simulink model "TBCC_Dyn_Template"  (Simulink 10.0)
settings: Solver=ode4  StartTime=0.0  StopTime=MWS.in.SimTime  FixedStep=MWS.Solve.T  RelTol=1e-3  EnableMultiTasking=on
undefined symbols (not defined in the file or in its folder): stripchar_TMATS
undefined symbols (not defined in the file): MWS
libraries: Lib_Solve_ModelSource_TMATS x2, Lib_Turbo_Ambient_TMATS x1, Lib_Turbo_Burner_TMATS x1, Lib_Turbo_Compressor_TMATS x1, Lib_Turbo_Duct_TMATS x1, Lib_Turbo_Inlet_TMATS x1, Lib_Turbo_Nozzle_TMATS x1, Lib_Turbo_Shaft_TMATS x1, Lib_Turbo_Turbine_TMATS x1, Lib_Solve_IterNRSolverJC_TMATS x1, Lib_Cntrl_FirstOrderSensor_TMATS x1, Lib_Solve_OuterLoopIntegrator_TMATS x1
CloseFcn:
  | run(strcat(MWS.top_level, filesep,'GasTurbine_Dyn_Example_cleanup'))
settings Model: Creator=jwchapm2  LastModifiedBy=Administrator
settings DataIOCC: LimitDataPoints=on  SignalLoggingName=SimulationOutput
settings OptimizationCC: BlockReduction=off  DefaultParameterBehavior=Inlined  BufferReuse=off  ExpressionDepthLimit=2147483647
settings DebuggingCC: SolverPrmCheckMsg=warning  StateNameClashWarn=warning
settings GRTTargetCC: GeneratePreprocessorConditionals=Disable all  CombineOutputUpdateFcns=on  GRTInterface=off
settings ConfigComp: CovExternalEMLEnable=off

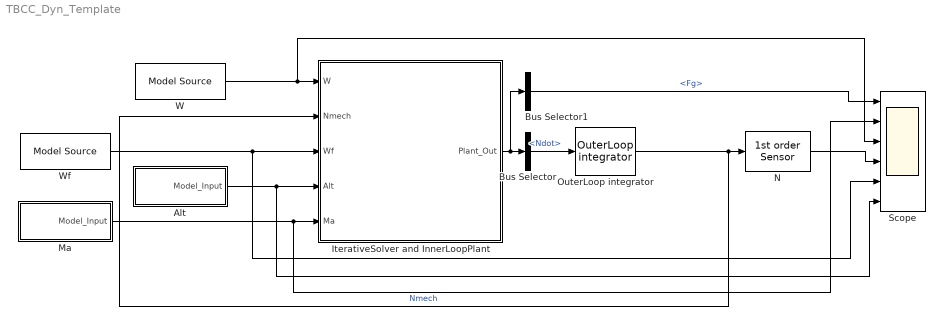
== system TBCC_Dyn_Template ==
  Alt : Subsystem  AncestorBlock=Lib_Solve_ModelSource_TMATS/Model Source  mask(T-MATS: Model Source Library Block){T_vec_M=MWS.in.t_vec, input_array_M=MWS.in.Alt}
      mask prompts: T_vec_M "T_vec_M - Time Vector (x-axis)"; input_array_M "input_array_M - Input Array 1-D ( f(Time))"
      mask help:
      | This block sets up the interface to change simulation variable dynamically.
      | Enter an input vector and time vector to allocate when each element
      | of the intput vector will occur.
      mask Help: web(which('Solver_TMATS_MS.html'),'-helpbrowser')
  Bus Selector : BusSelector  OutputSignals=PlantBus.Ndot
  Bus Selector1 : BusSelector  OutputSignals=PlantBus.Fg
  IterativeSolver and InnerLoopPlant : Subsystem
  Ma : Subsystem  AncestorBlock=Lib_Solve_ModelSource_TMATS/Model Source  mask(T-MATS: Model Source Library Block){T_vec_M=MWS.in.t_vec, input_array_M=MWS.in.Alt}
      mask prompts: T_vec_M "T_vec_M - Time Vector (x-axis)"; input_array_M "input_array_M - Input Array 1-D ( f(Time))"
      mask help:
      | This block sets up the interface to change simulation variable dynamically.
      | Enter an input vector and time vector to allocate when each element
      | of the intput vector will occur.
      mask Help: web(which('Solver_TMATS_MS.html'),'-helpbrowser')
  N : Lib_Cntrl_FirstOrderSensor_TMATS/1st order  Sensor  IC_M=MWS.Solve.N_IC  Sen_Max_M=20000  Sen_Min_M=0  Gain_M=1  Tau_M=0.05  GN_EN_M=off  GN_NST_M=MWS.Solve.T  GN_C_M=1  GN_MinNoise_M=0.3  F_Gain_M=1  F_Drift_M=0
  OuterLoop integrator : Lib_Solve_OuterLoopIntegrator_TMATS/OuterLoop integrator  OL_IC_M=MWS.Solve.N_IC
  Scope : Scope  NumInputPorts=6
  W : Lib_Solve_ModelSource_TMATS/Model Source  T_vec_M=MWS.in.t_vec  input_array_M=MWS.in.Alt
  Wf : Lib_Solve_ModelSource_TMATS/Model Source  T_vec_M=MWS.in.t_vec  input_array_M=MWS.in.Wf
  wires:
  IterativeSolver and InnerLoopPlant/1(Plant_Out) -> Bus Selector1/1, Bus Selector/1
  Bus Selector/1 -> OuterLoop integrator/1  "<Ndot>"
  OuterLoop integrator/1 -> N/1, IterativeSolver and InnerLoopPlant/2(Nmech)  "Nmech"
  Alt/1(Model_Input) -> Scope/6, IterativeSolver and InnerLoopPlant/4(Alt)
  Wf/1 -> Scope/5, IterativeSolver and InnerLoopPlant/3(Wf)
  W/1 -> Scope/3, IterativeSolver and InnerLoopPlant/1(W)
  Bus Selector1/1 -> Scope/1  "<Fg>"
  Ma/1(Model_Input) -> Scope/2, IterativeSolver and InnerLoopPlant/5(Ma)
  N/1 -> Scope/4

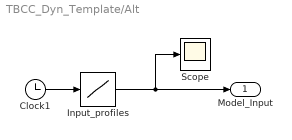
== system TBCC_Dyn_Template/Alt ==
  Clock1 : Clock
      settings: Decimation=100
  Input_profiles : Lookup  InputValues=T_vec_M  Table=input_array_M
  Scope : Scope
  Model_Input : Outport
  wires:
  Clock1/1 -> Input_profiles/1
  Input_profiles/1 -> Scope/1, Model_Input/1

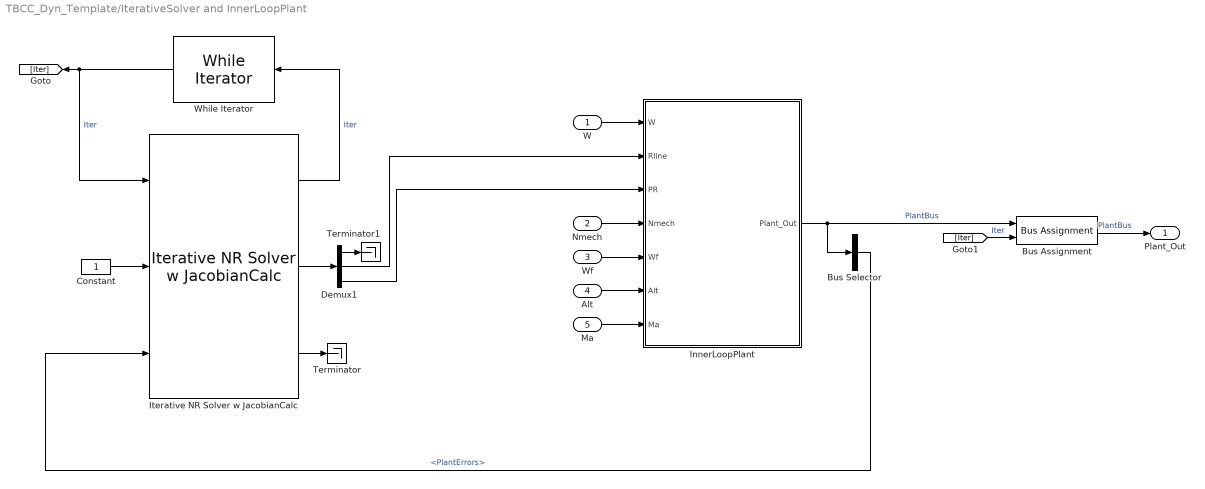
== system TBCC_Dyn_Template/IterativeSolver and InnerLoopPlant ==
  W : Inport
  Nmech : Inport  Port=2
  Wf : Inport  Port=3
  Alt : Inport  Port=4
  Ma : Inport  Port=5
  Bus Assignment : BusAssignment  AssignedSignals=PlantBus.Iter
  Bus Selector : BusSelector  OutputSignals=PlantErrors
  Constant : Constant
  Demux1 : Demux  Outputs=3
  InnerLoopPlant : Subsystem
  Iterative NR Solver w JacobianCalc : Lib_Solve_IterNRSolverJC_TMATS/Iterative NR Solver w JacobianCalc  SJac_Per_M=MWS.Solve.J_Calc_Per  SNR_IC_M=MWS.Solve.NR_IC  SNR_DX_M=MWS.Solve.NR_dx  SNR_Mx_M=100000  SNR_Mn_M=0.0001  SJacobianAttempts_M=MWS.Solve.NR_Jac_Re  Cond_Limits_M=MWS.Solve.C_Lim
  Terminator : Terminator
  Terminator1 : Terminator
  While Iterator : WhileIterator  MaxIters=MWS.Solve.Max_Iter  WhileBlockType=do-while  ShowIterationPort=on
  Plant_Out : Outport
  wires:
  Bus Selector/1 -> Iterative NR Solver w JacobianCalc/3  "<PlantErrors>"
  While Iterator/1 -> [Iter], Iterative NR Solver w JacobianCalc/1  "Iter"
  InnerLoopPlant/1(Plant_Out) -> Bus Selector/1, Bus Assignment/1  "PlantBus"
  Iterative NR Solver w JacobianCalc/1 -> While Iterator/1  "Iter"
  Iterative NR Solver w JacobianCalc/3 -> Terminator/1
  Constant/1 -> Iterative NR Solver w JacobianCalc/2
  [Iter] -> Bus Assignment/2  "Iter"
  Bus Assignment/1 -> Plant_Out/1  "PlantBus"
  W/1 -> InnerLoopPlant/1(W)
  Demux1/2 -> InnerLoopPlant/2(Rline)
  Demux1/3 -> InnerLoopPlant/3(PR)
  Iterative NR Solver w JacobianCalc/2 -> Demux1/1
  Demux1/1 -> Terminator1/1
  Nmech/1 -> InnerLoopPlant/4(Nmech)
  Wf/1 -> InnerLoopPlant/5(Wf)
  Alt/1 -> InnerLoopPlant/6(Alt)
  Ma/1 -> InnerLoopPlant/7(Ma)

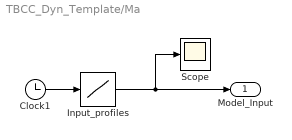
== system TBCC_Dyn_Template/Ma ==
  Clock1 : Clock
      settings: Decimation=100
  Input_profiles : Lookup  InputValues=T_vec_M  Table=input_array_M
  Scope : Scope
  Model_Input : Outport
  wires:
  Clock1/1 -> Input_profiles/1
  Input_profiles/1 -> Scope/1, Model_Input/1

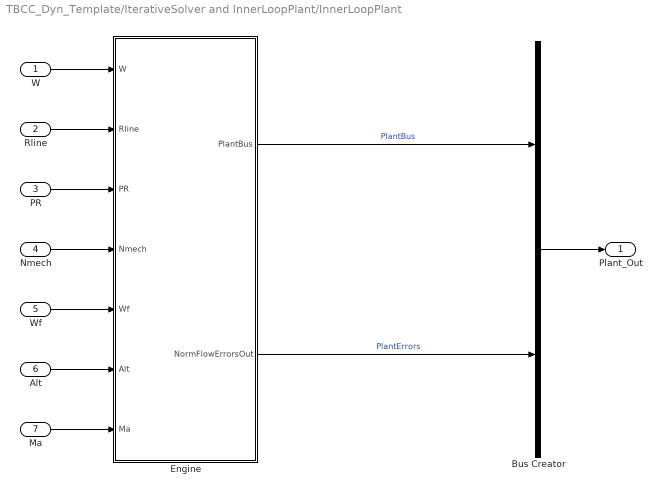
== system TBCC_Dyn_Template/IterativeSolver and InnerLoopPlant/InnerLoopPlant ==
  W : Inport
  Rline : Inport  Port=2
  PR : Inport  Port=3
  Nmech : Inport  Port=4
  Wf : Inport  Port=5
  Alt : Inport  Port=6
  Ma : Inport  Port=7
  Bus Creator : BusCreator  Inputs=2
  Engine : Subsystem
  Plant_Out : Outport
  wires:
  Engine/1(PlantBus) -> Bus Creator/1  "PlantBus"
  Engine/2(NormFlowErrorsOut) -> Bus Creator/2  "PlantErrors"
  Bus Creator/1 -> Plant_Out/1
  Wf/1 -> Engine/5(Wf)
  Nmech/1 -> Engine/4(Nmech)
  Alt/1 -> Engine/6(Alt)
  W/1 -> Engine/1(W)
  Rline/1 -> Engine/2(Rline)
  PR/1 -> Engine/3(PR)
  Ma/1 -> Engine/7(Ma)

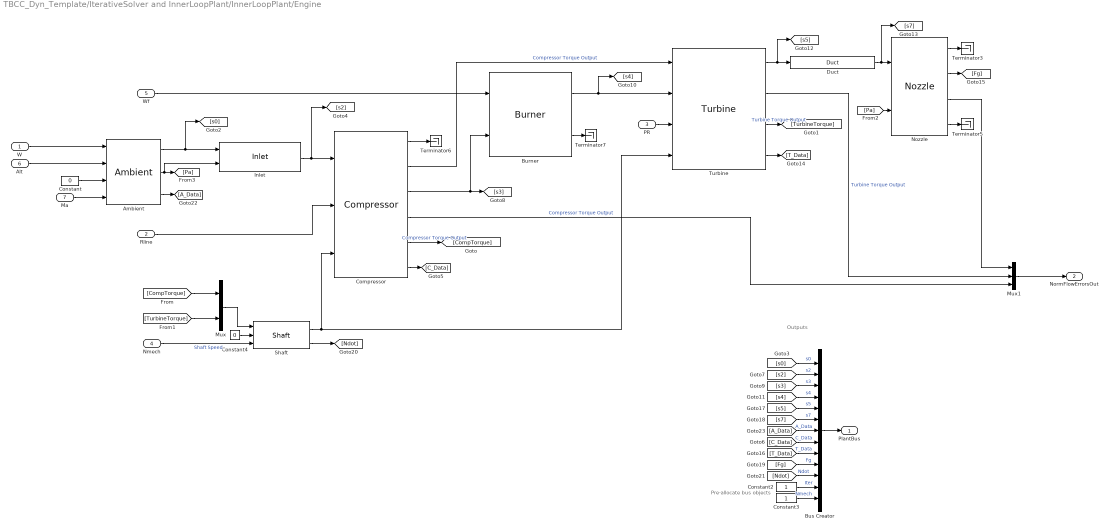
== system TBCC_Dyn_Template/IterativeSolver and InnerLoopPlant/InnerLoopPlant/Engine ==
  note: Pre-allocate bus objects
  note: Outputs
  W : Inport
  Rline : Inport  Port=2
  PR : Inport  Port=3
  Nmech : Inport  Port=4
  Wf : Inport  Port=5
  Alt : Inport  Port=6
  Ma : Inport  Port=7
  Ambient : Lib_Turbo_Ambient_TMATS/Ambient  X_A_AltVec_M=5000*[-1 0 1 2 3 4 5 6 7 8 9 10 12 14 16]  T_A_TsVec_M=[536.51 518.67 500.84 483.03 465.22 447.41 429.62 411.84 394.06 389.97 389.97 389.97 389.97 392.25 397.69]  T_A_PsVec_M=[17.554 14.696 12.228 10.108 8.297 6.759 5.461 4.373 3.468 2.73 2.149 1.692 1.049 0.651 0.406]  AFARc_M=0  X_A_FARVec_M=[0; 0.0050; 0.0100; 0.0150; 0.0200; 0.0250; 0.0300]  T_A_RtArray_M="[0.0686;    0.0686;    0.0686;    0.0686;    0.0686;    0.0686;    0.0686]"  Y_A_TVec_M=[300 10000]  T_A_gammaArray_M=[ 1.4 1.4 1.4 1.4 1.4 1.4 1.4; 1.4 1.4 1.4 1.4 1.4 1.4 1.4]
  Burner : Lib_Turbo_Burner_TMATS/Burner  LHVEn_M=on  LHV_M=MWS.Burner.LHV  Eff_M=1  hFuel_M=-1200  dPnormBurner_M=MWS.Burner.dP
  Bus Creator : BusCreator  Inputs=13
  Compressor : Lib_Turbo_Compressor_TMATS/Compressor  X_C_RlineVec_M=MWS.HPC.RlineVec  Z_C_AlphaVec_M=1  Y_C_Map_NcVec_M=MWS.HPC.NcVec  T_C_Map_WcArray_M=MWS.HPC.WcArray  T_C_Map_PRArray_M=MWS.HPC.PRArray  T_C_Map_EffArray_M=MWS.HPC.EffArray  s_C_Nc_M=MWS.HPC.s_Nc  s_C_Wc_M=MWS.HPC.s_Wc  s_C_PR_M=MWS.HPC.s_PR  s_C_Eff_M=MWS.HPC.s_eff  SL_M=off  Scale_M=none  CBLDEN_M=off  C_CBD_M=0  C_CBFht_M=0.5  C_CBFPt_M=0.5  FBLDEN_M=off  C_FBD_M=0  C_BFht_M=0.5  C_BFPt_M=0.5  DefSMEn_M=off  SMNEn_M=off  SRline_M=1  X_C_Map_WcSurgeVec_M=MWS.HPC.WcMapSurge  T_C_Map_PRSurgeVec_M=MWS.HPC.PRMapSurge  iDesign_M=2  NcDes_M=10000  EffDes_M=0.85  PRDes_M=20  RlineDes_M=2  FVar_M=strcat('iDes_',stripchar_TMATS(gcb),'.bin')  BlkNm_M=double(gcb)  HP_M=off
  Constant : Constant  Value=0
  Constant2 : Constant  OutDataTypeStr=int32
  Constant3 : Constant
  Constant4 : Constant  Value=0
  Duct : Lib_Turbo_Duct_TMATS/Duct  dP_M=MWS.Duct.dP
  Inlet : Lib_Turbo_Inlet_TMATS/Inlet  eRambase_M=MWS.Inlet.eRambase  X_eRamVec_M=[0 3]  T_eRamtbl_M=[1 1]
  Mux : Mux  Inputs=2
  Mux1 : Mux  Inputs=3
  Nozzle : Lib_Turbo_Nozzle_TMATS/Nozzle  SWType_M=Convergent  N_TArea_M=MWS.Noz.ATh  N_EArea_M=110.7  N_FL_M=MWS.Noz.LossPerc  X_N_TtVec2_M=MWS.Noz.TtVec  T_N_TGArray_M=MWS.Noz.TGArray  X_N_PEQPaVec_M=MWS.Noz.PeQPaVec  T_N_CdThArray_M=MWS.Noz.CdThArray  T_N_CvArray_M=MWS.Noz.CvArray  CfgEn_M=off  T_N_CfgArray_M=[1 1]  X_N_FARVec_M=MWS.Noz.FARVec  T_N_RtArray_M=MWS.Noz.RArray  Y_N_TtVec_M=MWS.Noz.TtVec  T_N_MAP_gammaArray_M=MWS.Noz.GArray  iDesign_M=2  WDes_M=100  FVar_M=strcat('iDes_',stripchar_TMATS(gcb),'.bin')
  Shaft : Lib_Turbo_Shaft_TMATS/Shaft  Shaft_Inertia_M=MWS.Shaft.N_I
  Terminator{3,5..7} (4 alike) : Terminator
  Turbine : Lib_Turbo_Turbine_TMATS/Turbine  X_T_Map_PRVec_M=MWS.HPT.PRVec  Y_T_Map_NcVec_M=MWS.HPT.NcVec  T_T_Map_WcArray_M=MWS.HPT.WcArray  T_T_Map_EffArray_M=MWS.HPT.EffArray  s_T_Nc_M=MWS.HPT.s_Nc  s_T_Wc_M=MWS.HPT.s_Wc  s_T_PR_M=MWS.HPT.s_PR  s_T_Eff_M=MWS.HPT.s_eff  ConfigNPSS_M=0  Scale_M=none  CFlwEn_M=off  T_CoolFlwPos_M=0  iDesign_M=2  NcDes_M=100  EffDes_M=0.9200  PRDes_M=5  NDes_M=10000  FVar_M=strcat('iDes_',stripchar_TMATS(gcb),'.bin')  BlkNm_M=double(gcb)  HP_M=off
  PlantBus : Outport
  NormFlowErrorsOut : Outport  Port=2
  wires:
  Compressor/6 -> [C_Data]
  Ambient/1 -> [s0], Inlet/1
  Duct/1 -> [s7], Nozzle/1
  Ambient/3 -> [A_Data]
  Ambient/2 -> [Pa], Inlet/2
  Ma/1 -> Ambient/4
  Constant/1 -> Ambient/3
  W/1 -> Ambient/1
  Nozzle/2 -> [Fg]
  Compressor/2 -> Turbine/1  "Compressor Torque Output"
  Compressor/1 -> Terminator6/1
  Shaft/1 -> Compressor/3, Turbine/4
  [TurbineTorque] -> Mux/2
  [CompTorque] -> Mux/1
  Turbine/3 -> [TurbineTorque]  "Turbine Torque Output"
  Compressor/5 -> [CompTorque]  "Compressor Torque Output"
  Mux/1 -> Shaft/1
  Shaft/2 -> [Ndot]
  Nmech/1 -> Shaft/3  "Shaft Speed"
  Inlet/1 -> [s2], Compressor/1
  Alt/1 -> Ambient/2
  Compressor/4 -> Mux1/3  "Compressor Torque Output"
  Turbine/2 -> Mux1/2  "Turbine Torque Output"
  Nozzle/4 -> Terminator5/1
  Nozzle/3 -> Mux1/1
  Nozzle/1 -> Terminator3/1
  Turbine/4 -> [T_Data]
  Mux1/1 -> NormFlowErrorsOut/1
  Rline/1 -> Compressor/2
  PR/1 -> Turbine/3
  Turbine/1 -> [s5], Duct/1
  Burner/1 -> [s4], Turbine/2
  [Pa] -> Nozzle/2
  Burner/2 -> Terminator7/1
  Wf/1 -> Burner/1
  Compressor/3 -> [s3], Burner/2
  [s0] -> Bus Creator/1  "s0"
  [s2] -> Bus Creator/2  "s2"
  [s3] -> Bus Creator/3  "s3"
  [s4] -> Bus Creator/4  "s4"
  [s5] -> Bus Creator/5  "s5"
  [s7] -> Bus Creator/6  "s7"
  [C_Data] -> Bus Creator/8  "C_Data"
  [T_Data] -> Bus Creator/9  "T_Data"
  [Fg] -> Bus Creator/10  "Fg"
  [Ndot] -> Bus Creator/11  "Ndot"
  Bus Creator/1 -> PlantBus/1
  [A_Data] -> Bus Creator/7  "A_Data"
  Constant2/1 -> Bus Creator/12  "Iter"
  Constant3/1 -> Bus Creator/13  "Nmech"
  Constant4/1 -> Shaft/2
